simulink model "Esempio7_s"  (R2021b)
settings: Solver=VariableStepAuto  StartTime=0.0  StopTime=10.0  RelTol=1e-3
undefined symbols (not defined in the file): A, B, C, D, e_i, hi, K1, L
settings Model: Creator=Steph  LastModifiedBy=Steph

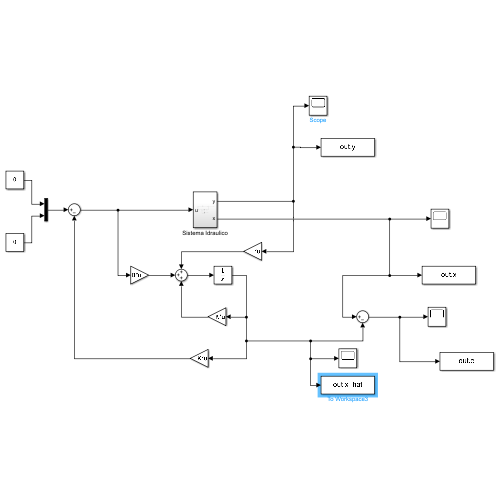
[thumbnail: Simulink's stored preview of the top-level diagram]
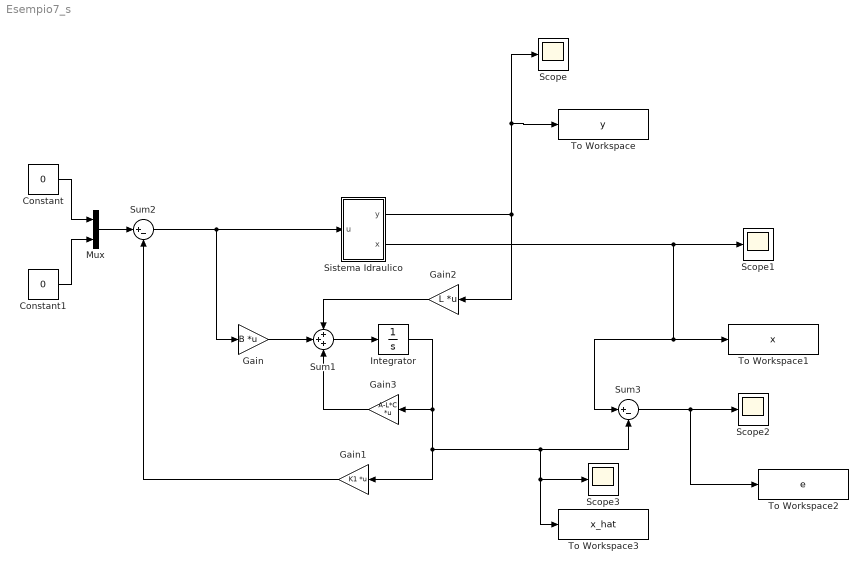
== system Esempio7_s ==
  Constant : Constant  Value=0
  Constant1 : Constant  Value=0
  Gain : Gain  Gain=B  Multiplication=Matrix(K*u)
  Gain1 : Gain  Gain=K1  Multiplication=Matrix(K*u)
  Gain2 : Gain  Gain=L  Multiplication=Matrix(K*u)
  Gain3 : Gain  Gain=A-L*C  Multiplication=Matrix(K*u)
  Integrator : Integrator  InitialCondition=hi-e_i
  Mux : Mux  Inputs=2
  Scope{,1..3} (4 alike) : Scope
  Sistema Idraulico : Subsystem
  Sum1 : Sum  Inputs=+++
  Sum2 : Sum  Inputs=|+-
  Sum3 : Sum  Inputs=|+-
  To Workspace : ToWorkspace  VariableName=y  SaveFormat=Timeseries  SampleTime=-1
  To Workspace1 : ToWorkspace  VariableName=x  SaveFormat=Timeseries  SampleTime=-1
  To Workspace2 : ToWorkspace  VariableName=e  SaveFormat=Timeseries  SampleTime=-1
  To Workspace3 : ToWorkspace  VariableName=x_hat  SaveFormat=Timeseries  SampleTime=-1
  wires:
  Sum2/1 -> Gain/1, Sistema Idraulico/1(u)
  Sistema Idraulico/1(y) -> Gain2/1, To Workspace/1, Scope/1
  Gain1/1 -> Sum2/2
  Integrator/1 -> To Workspace3/1, Scope3/1, Sum3/2, Gain1/1, Gain3/1
  Sum1/1 -> Integrator/1
  Gain2/1 -> Sum1/1
  Gain/1 -> Sum1/2
  Gain3/1 -> Sum1/3
  Sistema Idraulico/2(x) -> Sum3/1, To Workspace1/1, Scope1/1
  Constant/1 -> Mux/1
  Constant1/1 -> Mux/2
  Mux/1 -> Sum2/1
  Sum3/1 -> To Workspace2/1, Scope2/1

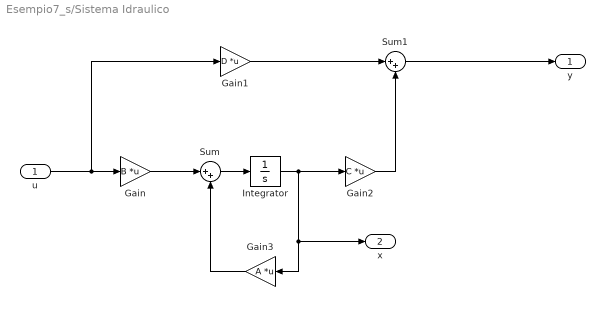
== system Esempio7_s/Sistema Idraulico ==
  u : Inport
  Gain : Gain  Gain=B  Multiplication=Matrix(K*u)
  Gain1 : Gain  Gain=D  Multiplication=Matrix(K*u)
  Gain2 : Gain  Gain=C  Multiplication=Matrix(K*u)
  Gain3 : Gain  Gain=A  Multiplication=Matrix(K*u)
  Integrator : Integrator  InitialCondition=hi
  Sum : Sum  Inputs=|++
  Sum1 : Sum  Inputs=|++
  y : Outport
  x : Outport  Port=2
  wires:
  Gain/1 -> Sum/1
  Gain2/1 -> Sum1/2
  Gain3/1 -> Sum/2
  Gain1/1 -> Sum1/1
  u/1 -> Gain1/1, Gain/1
  Integrator/1 -> Gain3/1, x/1, Gain2/1
  Sum/1 -> Integrator/1
  Sum1/1 -> y/1
